simulink model "sliding_mode_realpump_est"  (R2019a)
settings: Solver=VariableStepAuto  StartTime=0.0  StopTime=500  RelTol=1e-3
values from neighbouring files (symbols this model uses):
  Amatd = DSYS.A    [kalman_dynamic.m]
  Bmatd = DSYS.B    [kalman_dynamic.m]
  Cmatd = DSYS.C    [kalman_dynamic.m]
  P0 = 1*eye(2)    [kalman_dynamic.m]
  Ts = 1e-1    (= 0.1)    [kalman_dynamic.m]
  x0 = [h10; h20]    [kalman_dynamic.m]
undefined symbols (not defined in the file or in its folder): National_Instruments, PCI
libraries: sldrtlib x2, R7014E_lib x1, simulink x1
settings Model: Creator=marbla-6  LastModifiedBy=marbla-6
settings SolverCC: ZeroCrossAlgorithm=Adaptive
settings DebuggingCC: IgnoredZcDiagnostic=none

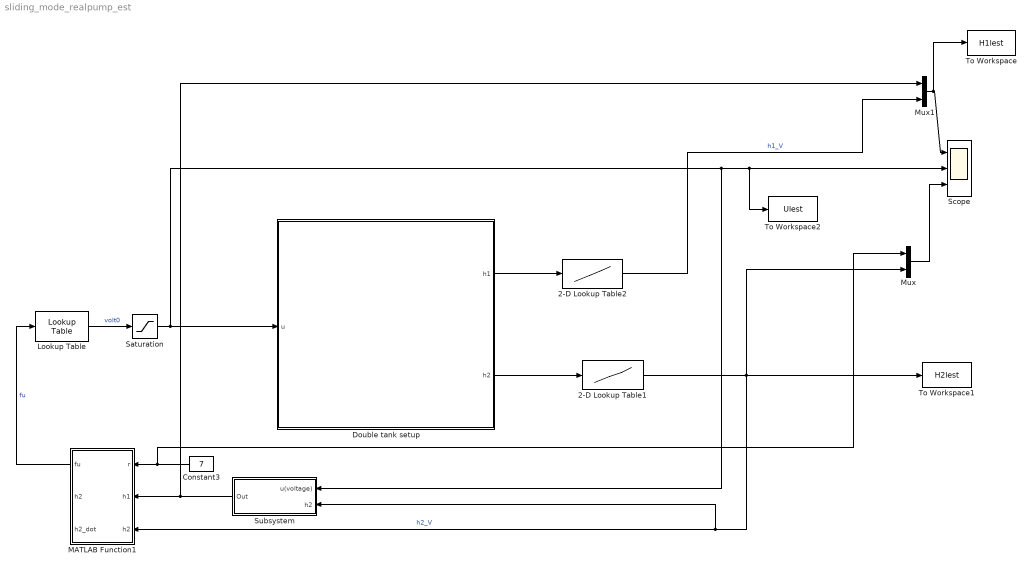
== system sliding_mode_realpump_est ==
  2-D Lookup Table1 : Lookup_n-D  NumberOfTableDimensions=1  BreakpointsForDimension1=x  BreakpointsForDimension2=[1:3]  Table=y  RndMeth=Simplest  InputSameDT=on  mask{x=[0.21,0.62,1.00,1.49,1.80,2.12,2.54,2.97,3.32,3.71,4.09,4.51,4.87,5.25,5.57,6.04,6.41,6.78,7.13,7.56,7.91,8.32,8.69,9.07,9.42,9.82,9.99], y=[2.50,3.00,3.50,4.00,4.50,5.00,5.50,6.00,6.50,7.00,7.50,8.00,8.50,9.00,9.50,10.00,10.50,11.00,11.50,12.00,12.50,13.00,13.50,14.00,14.50,15.00,15.50]}
      mask prompts: x "Values on x-axis"; y "Values on y-axis"
  2-D Lookup Table2 : Lookup_n-D  NumberOfTableDimensions=1  BreakpointsForDimension1=x  BreakpointsForDimension2=[1:3]  Table=y  RndMeth=Simplest  InputSameDT=on  mask{x=[0.21,0.62,1.00,1.49,1.80,2.12,2.54,2.97,3.32,3.71,4.09,4.51,4.87,5.25,5.57,6.04,6.41,6.78,7.13,7.56,7.91,8.32,8.69,9.07,9.42,9.82,9.99], y=[2.50,3.00,3.50,4.00,4.50,5.00,5.50,6.00,6.50,7.00,7.50,8.00,8.50,9.00,9.50,10.00,10.50,11.00,11.50,12.00,12.50,13.00,13.50,14.00,14.50,15.00,15.50]}
      mask prompts: x "Values on x-axis"; y "Values on y-axis"
  Constant3 : Constant  Value=7
  Double tank setup : Subsystem  AncestorBlock=R7014E_lib/Double tank setup  StopFcn=|  mask(Realtime interface for the tank process){ts=0.02, h1_ch=0, h2_ch=1, u_ch=0}
      | chn =get_param(gcb,'u_ch');                          
      | s = daq.createSession('ni');                         
      | channel = ['ao',chn];                                
      | s.addAnalogOutputChannel('Dev1', channel, 'Voltage');
      | x = zeros(5,1);                                      
      | s.queueOutputData(x);                                
      | lh = s.addlistener('DataRequired', ...               
      | @(src,event) src.queueOutputData(x));                
      | s.startBackground();                                 
      | s.wait();                                            
      | s.stop();                                            
      | delete(lh);                                          
      | clear chn;                                           
      | clear s;                                             
      | clear channel;                                       
      | clear lh;                                            
      | clear x;
      mask prompts: ts "Sample time"; h1_ch "A/D Channel for upper tank"; h2_ch "A/D Channel for lower tank"; u_ch "D/A Channel for pump"
      mask help:
      | This block represents the physical interface from the computer to the tank process.
      |
      | The input u is the voltage that is provided for the pump, the output h1 is the measured level in the upper tank in [V] and the output h2 is the
      | measured level in the lower tank in [V].
      |
      | You need to provide the sample rate at which the voltage to the pump is updated and the level measurements are sampled. The sample rate should not be less than 0.02 seconds.
      mask Display:
      | x=363;
      | y=381;
      | image(imread('tank_icon.jpg'));
      | text(250/x,309/y,'Sensor');
      | text(260/x,169/y,'Sensor');
      | text(335/x,289/y,'A');
      | text(351/x,283/y,'D');
      | text(335/x,100/y,'A');
      | text(351/x,95/y,'D');
      | text(22/x,187/y,'A');
      | text(5/x,195/y,'D');
      | text(225/x,278/y,'h_1','texmode','on');
      | text(225/x,146/y,'h_2','texmode','on');
      | text(300/x,270/y,sprintf('AI-%d',h1_ch));
      | text(300/x,80/y,sprintf('AI-%d',h2_ch));
      | text(40/x,173/y,sprintf('AO-%d',u_ch));
  Lookup Table : R7014E_lib/Lookup Table  x=[16.47,20.75,24.52,27.63,30.06,32.49,34.8,40.28,48.24,52.43]  y=[0.5,1,1.5,2,2.5,3,3.5,5,8,10]
  MATLAB Function1 : MATLAB Function  TreatAsAtomicUnit=on
  Mux : Mux  Inputs=2
  Mux1 : Mux  Inputs=2
  Saturation : Saturate  UpperLimit=10  LowerLimit=0
  Scope : Scope  NumInputPorts=3
  Subsystem : Subsystem
  To Workspace : ToWorkspace  VariableName=H1lest  SaveFormat=Timeseries  SampleTime=-1
  To Workspace1 : ToWorkspace  VariableName=H2lest  SaveFormat=Timeseries  SampleTime=-1
  To Workspace2 : ToWorkspace  VariableName=Ulest  SaveFormat=Timeseries  SampleTime=-1
  wires:
  Constant3/1 -> MATLAB Function1/1(r), Mux/1
  Lookup Table/1 -> Saturation/1  "volt0"
  Saturation/1 -> Double tank setup/1(u), Subsystem/1(u(voltage)), Scope/2, To Workspace2/1
  Double tank setup/1(h1) -> 2-D Lookup Table2/1
  2-D Lookup Table2/1 -> Mux1/2  "h1_V"
  Double tank setup/2(h2) -> 2-D Lookup Table1/1
  2-D Lookup Table1/1 -> To Workspace1/1, Mux/2, MATLAB Function1/3("h2 "), Subsystem/2(h2)  "h2_V"
  Mux/1 -> Scope/3
  Mux1/1 -> To Workspace/1, Scope/1
  Subsystem/1(Out) -> MATLAB Function1/2(h1), Mux1/1
  MATLAB Function1/1(fu) -> Lookup Table/1  "fu"

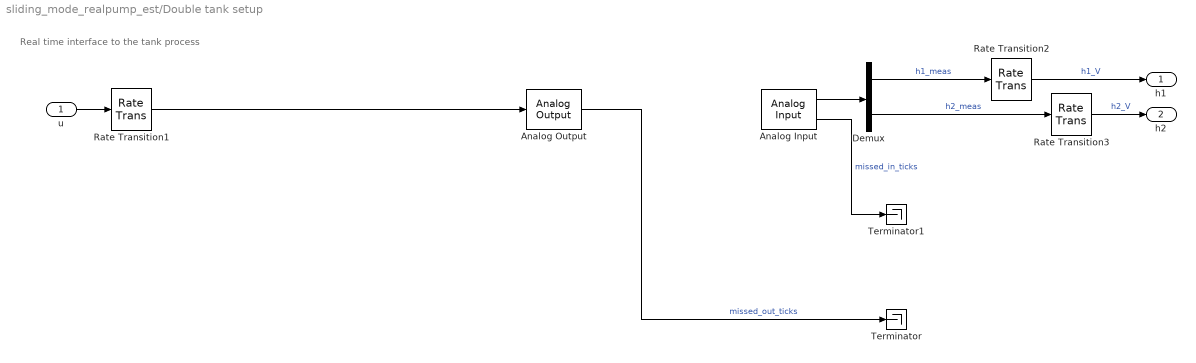
== system sliding_mode_realpump_est/Double tank setup ==
  note: Real time interface to the tank process
  u : Inport
  Analog Input : sldrtlib/Analog Input  SampleTime=ts  MaxMissedTicks=500000000  ShowMissedTicks=on  YieldWhenWaiting=off  DrvName=National_Instruments/PCI-6024E  DrvAddress=4294967295  DrvOptions=[0 0 0 0 0 0]  Channels=[h1_ch+1,h2_ch+1]  RangeMode=1  VoltRange=1  DataType=1
      settings: AttributesFormatString=National Instruments\nPCI-6024E [auto]  SourceProductName=Simulink Desktop Real-Time
  Analog Output : sldrtlib/Analog Output  SampleTime=ts  MaxMissedTicks=500000000  ShowMissedTicks=on  YieldWhenWaiting=off  DrvName=National_Instruments/PCI-6024E  DrvAddress=4294967295  DrvOptions=[0 0 0 0 0 0]  Channels=u_ch+1  RangeMode=1  VoltRange=1  InitialValue=0  FinalValue=0
      settings: AttributesFormatString=National Instruments\nPCI-6024E [auto]  SourceProductName=Simulink Desktop Real-Time
  Demux : Demux  Outputs=2
  Rate Transition1 : RateTransition  OutPortSampleTime=ts
  Rate Transition2 : RateTransition
  Rate Transition3 : RateTransition
  Terminator : Terminator
  Terminator1 : Terminator
  h1 : Outport
  h2 : Outport  Port=2
  wires:
  Rate Transition1/1 -> Analog Output/1
  Rate Transition3/1 -> h2/1  "h2_V"
  Rate Transition2/1 -> h1/1  "h1_V"
  Analog Input/2 -> Terminator1/1  "missed_in_ticks"
  Demux/2 -> Rate Transition3/1  "h2_meas"
  Demux/1 -> Rate Transition2/1  "h1_meas"
  Analog Input/1 -> Demux/1
  Analog Output/1 -> Terminator/1  "missed_out_ticks"
  u/1 -> Rate Transition1/1

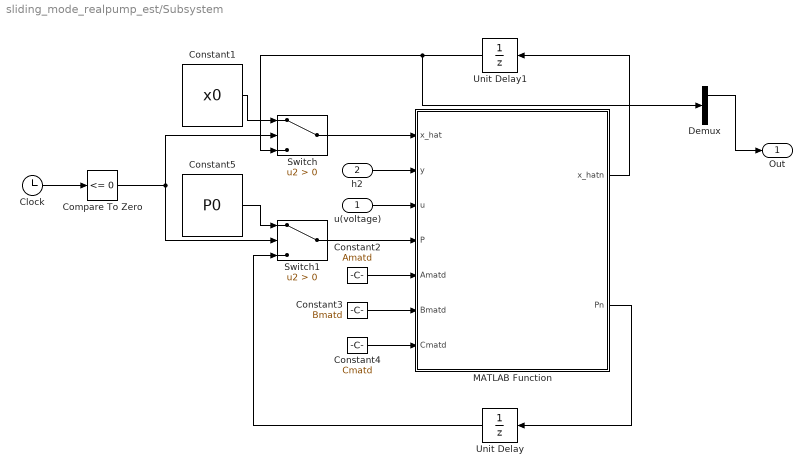
== system sliding_mode_realpump_est/Subsystem ==
  u(voltage) : Inport
  h2 : Inport  Port=2
  Clock : Clock
  Compare To Zero : simulink/Logic and Bit Operations/Compare To Zero  relop=<=  OutDataTypeStr=boolean
  Constant1 : Constant  Value=x0  VectorParams1D=off  SampleTime=Ts
  Constant2 : Constant  Value=Amatd  VectorParams1D=off  SampleTime=Ts
  Constant3 : Constant  Value=Bmatd  VectorParams1D=off  SampleTime=Ts
  Constant4 : Constant  Value=Cmatd  VectorParams1D=off  SampleTime=Ts
  Constant5 : Constant  Value=P0  VectorParams1D=off  SampleTime=Ts
  Demux : Demux  Outputs=2
  MATLAB Function : MATLAB Function  TreatAsAtomicUnit=on
  Switch : Switch  Criteria=u2 > Threshold
  Switch1 : Switch  Criteria=u2 > Threshold
  Unit Delay : UnitDelay  SampleTime=Ts  HasFrameUpgradeWarning=on
  Unit Delay1 : UnitDelay  SampleTime=Ts  HasFrameUpgradeWarning=on
  Out : Outport
  wires:
  h2/1 -> MATLAB Function/2(y)
  u(voltage)/1 -> MATLAB Function/3(u)
  Constant2/1 -> MATLAB Function/5(Amatd)
  Constant4/1 -> MATLAB Function/7(Cmatd)
  Constant3/1 -> MATLAB Function/6(Bmatd)
  MATLAB Function/2(Pn) -> Unit Delay/1
  Constant1/1 -> Switch/1
  Unit Delay1/1 -> Demux/1, Switch/3
  Unit Delay/1 -> Switch1/3
  Constant5/1 -> Switch1/1
  Clock/1 -> Compare To Zero/1
  Compare To Zero/1 -> Switch/2, Switch1/2
  Switch1/1 -> MATLAB Function/4(P)
  Switch/1 -> MATLAB Function/1(x_hat)
  MATLAB Function/1(x_hatn) -> Unit Delay1/1
  Demux/1 -> Out/1

== matlab function sliding_mode_realpump_est/Subsystem/MATLAB Function ==
  data: x_hat input; y input; u input; x_hatn output; P input; Pn output; Amatd input; Bmatd input; Cmatd input
function [x_hatn, Pn ] = fcn(x_hat, y, u, P, Amatd, Bmatd, Cmatd)

    Q = 40*eye(2);
    N = 1*eye(2);
    R = 10*eye(2);

    x_hatn = Amatd*x_hat + Bmatd*u;
    Pn = Amatd*P*Amatd' + N*Q*N';  

    K = (Pn*Cmatd')\(Cmatd*Pn*Cmatd' + R);
    y_til = y - Cmatd*x_hatn;
    x_hatn = x_hatn + K*[0; y_til];
    Pn = Pn - K*Cmatd'*Pn;
    
end

== matlab function sliding_mode_realpump_est/MATLAB Function1 ==
  data: r input; h1 input; fu output; h2 input; h2 output; h2_dot output
function [fu,h2, h2_dot ] = fcn(r, h1, h2)

    % h1, h2 are including outlet height
    
    a = 0.16;
    A = 33;
    g = 982;
    h0 = 3.2;
    
    mu = .17*10;
    p1 = 0.9;
    p2 = 0.1;
    p = [p1; p2];
    eps = 0.5;
    
    
    h2_dot = (a/A)*sqrt(2*g)*(sqrt(h1+h0)-sqrt(h2+h0)); 
    
    beta = [(a/(2*A^2))*sqrt((2*g)/(h1+h0));0]; %g(x)
    alpha = [-(a^2/A^2)*g*sqrt((h1+h0)/(h2+h0));h2_dot]; %f(x)

    h2 = h2 - r;
    sigma = p1*h2_dot + p2*h2;
    
    if abs(sigma) < eps
        ssat = sigma/eps;
    else
        ssat = sign(sigma);        
    end
    
    fu = (-p' * alpha) / (p'*beta) - (mu / (p'*beta)) * ssat;
    
end

%     l_1 = -p1-p2;
%     l_2 = p1*p2;
%     
%     L = [l_2 l_1];
%     Lr = l_2;
%     h_2d = (a/A) * (sqrt(2*g*h1) - sqrt(2*g*h2)) %f(x)
%     alpha = -(a^2/A^2)*g*sqrt((h1+h0)/(h2+h0));
%     beta = (a/(2*A^2))*sqrt((2*g)/(h1+h0));
%    
%     
%     x1 = h2;
%     x2 = h2_dot;  
%     x = [x1; x2];
%     
%   
%     fu = (1/beta)*(-L*x+Lr*r-alpha);
%
